simulink model "adcddcxaui_100"  (Simulink 6.2)
settings: Solver=ode45  StartTime=0.0  StopTime=1000  RelTol=1e-3
undefined symbols (not defined in the file): BitWidth
libraries: xbsIndex_r3 x358, casper_library x26, xps_library x12
(part 2 of 4)

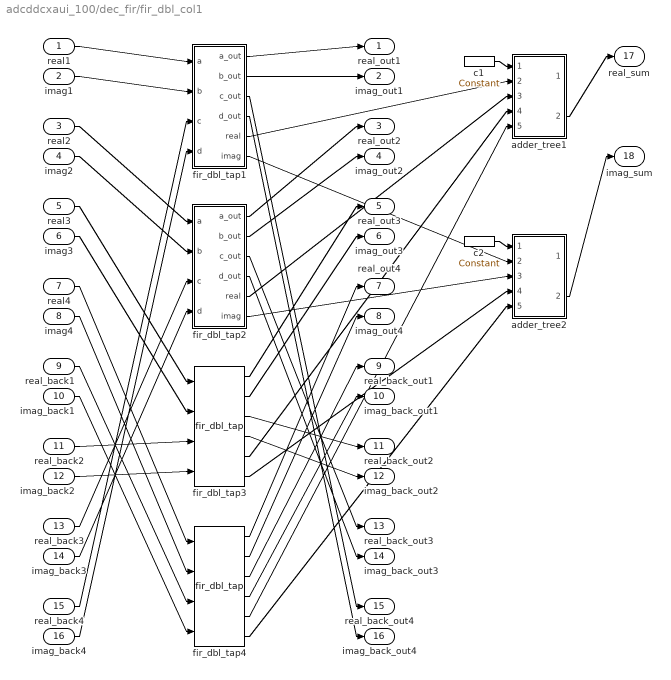
== system adcddcxaui_100/dec_fir/fir_dbl_col1 ==
  real1 : Inport  Port=1  LatchInput=off
  imag1 : Inport  Port=2  LatchInput=off
  real2 : Inport  Port=3  LatchInput=off
  imag2 : Inport  Port=4  LatchInput=off
  real3 : Inport  Port=5  LatchInput=off
  imag3 : Inport  Port=6  LatchInput=off
  real4 : Inport  Port=7  LatchInput=off
  imag4 : Inport  Port=8  LatchInput=off
  real_back1 : Inport  Port=9  LatchInput=off
  imag_back1 : Inport  Port=10  LatchInput=off
  real_back2 : Inport  Port=11  LatchInput=off
  imag_back2 : Inport  Port=12  LatchInput=off
  real_back3 : Inport  Port=13  LatchInput=off
  imag_back3 : Inport  Port=14  LatchInput=off
  real_back4 : Inport  Port=15  LatchInput=off
  imag_back4 : Inport  Port=16  LatchInput=off
  adder_tree1 : Subsystem  AncestorBlock=casper_library/Misc/adder_tree  mask(adder_tree){n_inputs=4, latency=2}
      mask prompts: n_inputs "Number of Inputs"; latency "Add Latency"
      mask help: Sums all inputs using a tree of adds and delays.
      mask init:
      | adder_tree_init(gcb, ...
      |     'n_inputs', n_inputs, ...
      |     'latency', latency);
      settings: AttributesFormatString=latency 4
      mask Help: eval('xlWeb([getenv(''MLIB_ROOT''), ''\doc\html\sp_adder_tree\sp_adder_tree.html''])')
  adder_tree2 : Subsystem  AncestorBlock=casper_library/Misc/adder_tree  mask(adder_tree){n_inputs=4, latency=2}
      mask prompts: n_inputs "Number of Inputs"; latency "Add Latency"
      mask help: Sums all inputs using a tree of adds and delays.
      mask init:
      | adder_tree_init(gcb, ...
      |     'n_inputs', n_inputs, ...
      |     'latency', latency);
      settings: AttributesFormatString=latency 4
      mask Help: eval('xlWeb([getenv(''MLIB_ROOT''), ''\doc\html\sp_adder_tree\sp_adder_tree.html''])')
  c1 : xbsIndex_r3/Constant  const=1  equ=P=C  arith_type=Unsigned  n_bits=1  bin_pt=0  opselect=C  inp2=PCIN>>17  opr=+  inp1=P  carry=CIN  iostate=0  explicit_period=on  period=1  dbl_ovrd=off
  c2 : xbsIndex_r3/Constant  const=1  equ=P=C  arith_type=Unsigned  n_bits=1  bin_pt=0  opselect=C  inp2=PCIN>>17  opr=+  inp1=P  carry=CIN  iostate=0  explicit_period=on  period=1  dbl_ovrd=off
  fir_dbl_tap1 : Subsystem  AncestorBlock=casper_library/Downconverter/fir_dbl_tap  mask(fir_dbl_tap){factor=-6.8471e-006, add_latency=2, mult_latency=2}
      mask prompts: add_latency "Add latency"; mult_latency "Mult latency"
  fir_dbl_tap2 : Subsystem  AncestorBlock=casper_library/Downconverter/fir_dbl_tap  mask(fir_dbl_tap){factor=-6.7515e-006, add_latency=2, mult_latency=2}
      mask prompts: add_latency "Add latency"; mult_latency "Mult latency"
  fir_dbl_tap3 : casper_library/Downconverter/fir_dbl_tap  factor=-1.9679e-006  add_latency=2  mult_latency=2
      link override Constant: equ=P=C
  fir_dbl_tap4 : casper_library/Downconverter/fir_dbl_tap  factor=-2.3202e-007  add_latency=2  mult_latency=2
      link override Constant: equ=P=C
  real_out1 : Outport
  imag_out1 : Outport  Port=2
  real_out2 : Outport  Port=3
  imag_out2 : Outport  Port=4
  real_out3 : Outport  Port=5
  imag_out3 : Outport  Port=6
  real_out4 : Outport  Port=7
  imag_out4 : Outport  Port=8
  real_back_out1 : Outport  Port=9
  imag_back_out1 : Outport  Port=10
  real_back_out2 : Outport  Port=11
  imag_back_out2 : Outport  Port=12
  real_back_out3 : Outport  Port=13
  imag_back_out3 : Outport  Port=14
  real_back_out4 : Outport  Port=15
  imag_back_out4 : Outport  Port=16
  real_sum : Outport  Port=17
  imag_sum : Outport  Port=18
  wires:
  c1/1 -> adder_tree1/1(sync)
  c2/1 -> adder_tree2/1(sync)
  adder_tree1/2(dout) -> real_sum/1
  adder_tree2/2(dout) -> imag_sum/1
  real1/1 -> fir_dbl_tap1/1(a)
  imag1/1 -> fir_dbl_tap1/2(b)
  real_back4/1 -> fir_dbl_tap1/3(c)
  imag_back4/1 -> fir_dbl_tap1/4(d)
  fir_dbl_tap1/1(a_out) -> real_out1/1
  fir_dbl_tap1/2(b_out) -> imag_out1/1
  fir_dbl_tap1/3(c_out) -> real_back_out4/1
  fir_dbl_tap1/4(d_out) -> imag_back_out4/1
  fir_dbl_tap1/5(real) -> adder_tree1/2(din1)
  fir_dbl_tap1/6(imag) -> adder_tree2/2(din1)
  real2/1 -> fir_dbl_tap2/1(a)
  imag2/1 -> fir_dbl_tap2/2(b)
  real_back3/1 -> fir_dbl_tap2/3(c)
  imag_back3/1 -> fir_dbl_tap2/4(d)
  fir_dbl_tap2/1(a_out) -> real_out2/1
  fir_dbl_tap2/2(b_out) -> imag_out2/1
  fir_dbl_tap2/3(c_out) -> real_back_out3/1
  fir_dbl_tap2/4(d_out) -> imag_back_out3/1
  fir_dbl_tap2/5(real) -> adder_tree1/3(din2)
  fir_dbl_tap2/6(imag) -> adder_tree2/3(din2)
  real3/1 -> fir_dbl_tap3/1
  imag3/1 -> fir_dbl_tap3/2
  real_back2/1 -> fir_dbl_tap3/3
  imag_back2/1 -> fir_dbl_tap3/4
  fir_dbl_tap3/1 -> real_out3/1
  fir_dbl_tap3/2 -> imag_out3/1
  fir_dbl_tap3/3 -> real_back_out2/1
  fir_dbl_tap3/4 -> imag_back_out2/1
  fir_dbl_tap3/5 -> adder_tree1/4(din3)
  fir_dbl_tap3/6 -> adder_tree2/4(din3)
  real4/1 -> fir_dbl_tap4/1
  imag4/1 -> fir_dbl_tap4/2
  real_back1/1 -> fir_dbl_tap4/3
  imag_back1/1 -> fir_dbl_tap4/4
  fir_dbl_tap4/1 -> real_out4/1
  fir_dbl_tap4/2 -> imag_out4/1
  fir_dbl_tap4/3 -> real_back_out1/1
  fir_dbl_tap4/4 -> imag_back_out1/1
  fir_dbl_tap4/5 -> adder_tree1/5(din4)
  fir_dbl_tap4/6 -> adder_tree2/5(din4)

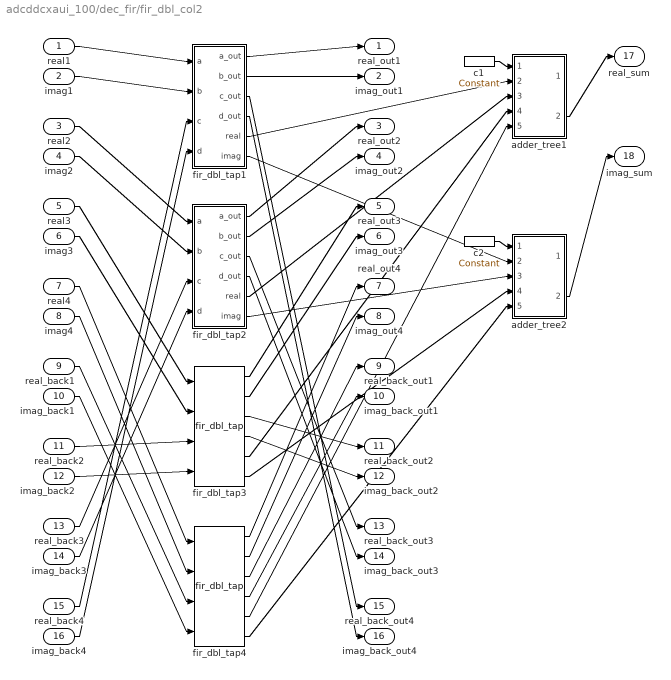
== system adcddcxaui_100/dec_fir/fir_dbl_col2 ==
  real1 : Inport  Port=1  LatchInput=off
  imag1 : Inport  Port=2  LatchInput=off
  real2 : Inport  Port=3  LatchInput=off
  imag2 : Inport  Port=4  LatchInput=off
  real3 : Inport  Port=5  LatchInput=off
  imag3 : Inport  Port=6  LatchInput=off
  real4 : Inport  Port=7  LatchInput=off
  imag4 : Inport  Port=8  LatchInput=off
  real_back1 : Inport  Port=9  LatchInput=off
  imag_back1 : Inport  Port=10  LatchInput=off
  real_back2 : Inport  Port=11  LatchInput=off
  imag_back2 : Inport  Port=12  LatchInput=off
  real_back3 : Inport  Port=13  LatchInput=off
  imag_back3 : Inport  Port=14  LatchInput=off
  real_back4 : Inport  Port=15  LatchInput=off
  imag_back4 : Inport  Port=16  LatchInput=off
  adder_tree1 : Subsystem  AncestorBlock=casper_library/Misc/adder_tree  mask(adder_tree){n_inputs=4, latency=2}
      mask prompts: n_inputs "Number of Inputs"; latency "Add Latency"
      mask help: Sums all inputs using a tree of adds and delays.
      mask init:
      | adder_tree_init(gcb, ...
      |     'n_inputs', n_inputs, ...
      |     'latency', latency);
      settings: AttributesFormatString=latency 4
      mask Help: eval('xlWeb([getenv(''MLIB_ROOT''), ''\doc\html\sp_adder_tree\sp_adder_tree.html''])')
  adder_tree2 : Subsystem  AncestorBlock=casper_library/Misc/adder_tree  mask(adder_tree){n_inputs=4, latency=2}
      mask prompts: n_inputs "Number of Inputs"; latency "Add Latency"
      mask help: Sums all inputs using a tree of adds and delays.
      mask init:
      | adder_tree_init(gcb, ...
      |     'n_inputs', n_inputs, ...
      |     'latency', latency);
      settings: AttributesFormatString=latency 4
      mask Help: eval('xlWeb([getenv(''MLIB_ROOT''), ''\doc\html\sp_adder_tree\sp_adder_tree.html''])')
  c1 : xbsIndex_r3/Constant  const=1  equ=P=C  arith_type=Unsigned  n_bits=1  bin_pt=0  opselect=C  inp2=PCIN>>17  opr=+  inp1=P  carry=CIN  iostate=0  explicit_period=on  period=1  dbl_ovrd=off
  c2 : xbsIndex_r3/Constant  const=1  equ=P=C  arith_type=Unsigned  n_bits=1  bin_pt=0  opselect=C  inp2=PCIN>>17  opr=+  inp1=P  carry=CIN  iostate=0  explicit_period=on  period=1  dbl_ovrd=off
  fir_dbl_tap1 : Subsystem  AncestorBlock=casper_library/Downconverter/fir_dbl_tap  mask(fir_dbl_tap){factor=7.4933e-005, add_latency=2, mult_latency=2}
      mask prompts: add_latency "Add latency"; mult_latency "Mult latency"
  fir_dbl_tap2 : Subsystem  AncestorBlock=casper_library/Downconverter/fir_dbl_tap  mask(fir_dbl_tap){factor=0.00010979, add_latency=2, mult_latency=2}
      mask prompts: add_latency "Add latency"; mult_latency "Mult latency"
  fir_dbl_tap3 : casper_library/Downconverter/fir_dbl_tap  factor=6.3269e-005  add_latency=2  mult_latency=2
      link override Constant: equ=P=C
  fir_dbl_tap4 : casper_library/Downconverter/fir_dbl_tap  factor=1.4095e-005  add_latency=2  mult_latency=2
      link override Constant: equ=P=C
  real_out1 : Outport
  imag_out1 : Outport  Port=2
  real_out2 : Outport  Port=3
  imag_out2 : Outport  Port=4
  real_out3 : Outport  Port=5
  imag_out3 : Outport  Port=6
  real_out4 : Outport  Port=7
  imag_out4 : Outport  Port=8
  real_back_out1 : Outport  Port=9
  imag_back_out1 : Outport  Port=10
  real_back_out2 : Outport  Port=11
  imag_back_out2 : Outport  Port=12
  real_back_out3 : Outport  Port=13
  imag_back_out3 : Outport  Port=14
  real_back_out4 : Outport  Port=15
  imag_back_out4 : Outport  Port=16
  real_sum : Outport  Port=17
  imag_sum : Outport  Port=18
  wires:
  c1/1 -> adder_tree1/1(sync)
  c2/1 -> adder_tree2/1(sync)
  adder_tree1/2(dout) -> real_sum/1
  adder_tree2/2(dout) -> imag_sum/1
  real1/1 -> fir_dbl_tap1/1(a)
  imag1/1 -> fir_dbl_tap1/2(b)
  real_back4/1 -> fir_dbl_tap1/3(c)
  imag_back4/1 -> fir_dbl_tap1/4(d)
  fir_dbl_tap1/1(a_out) -> real_out1/1
  fir_dbl_tap1/2(b_out) -> imag_out1/1
  fir_dbl_tap1/3(c_out) -> real_back_out4/1
  fir_dbl_tap1/4(d_out) -> imag_back_out4/1
  fir_dbl_tap1/5(real) -> adder_tree1/2(din1)
  fir_dbl_tap1/6(imag) -> adder_tree2/2(din1)
  real2/1 -> fir_dbl_tap2/1(a)
  imag2/1 -> fir_dbl_tap2/2(b)
  real_back3/1 -> fir_dbl_tap2/3(c)
  imag_back3/1 -> fir_dbl_tap2/4(d)
  fir_dbl_tap2/1(a_out) -> real_out2/1
  fir_dbl_tap2/2(b_out) -> imag_out2/1
  fir_dbl_tap2/3(c_out) -> real_back_out3/1
  fir_dbl_tap2/4(d_out) -> imag_back_out3/1
  fir_dbl_tap2/5(real) -> adder_tree1/3(din2)
  fir_dbl_tap2/6(imag) -> adder_tree2/3(din2)
  real3/1 -> fir_dbl_tap3/1
  imag3/1 -> fir_dbl_tap3/2
  real_back2/1 -> fir_dbl_tap3/3
  imag_back2/1 -> fir_dbl_tap3/4
  fir_dbl_tap3/1 -> real_out3/1
  fir_dbl_tap3/2 -> imag_out3/1
  fir_dbl_tap3/3 -> real_back_out2/1
  fir_dbl_tap3/4 -> imag_back_out2/1
  fir_dbl_tap3/5 -> adder_tree1/4(din3)
  fir_dbl_tap3/6 -> adder_tree2/4(din3)
  real4/1 -> fir_dbl_tap4/1
  imag4/1 -> fir_dbl_tap4/2
  real_back1/1 -> fir_dbl_tap4/3
  imag_back1/1 -> fir_dbl_tap4/4
  fir_dbl_tap4/1 -> real_out4/1
  fir_dbl_tap4/2 -> imag_out4/1
  fir_dbl_tap4/3 -> real_back_out1/1
  fir_dbl_tap4/4 -> imag_back_out1/1
  fir_dbl_tap4/5 -> adder_tree1/5(din4)
  fir_dbl_tap4/6 -> adder_tree2/5(din4)

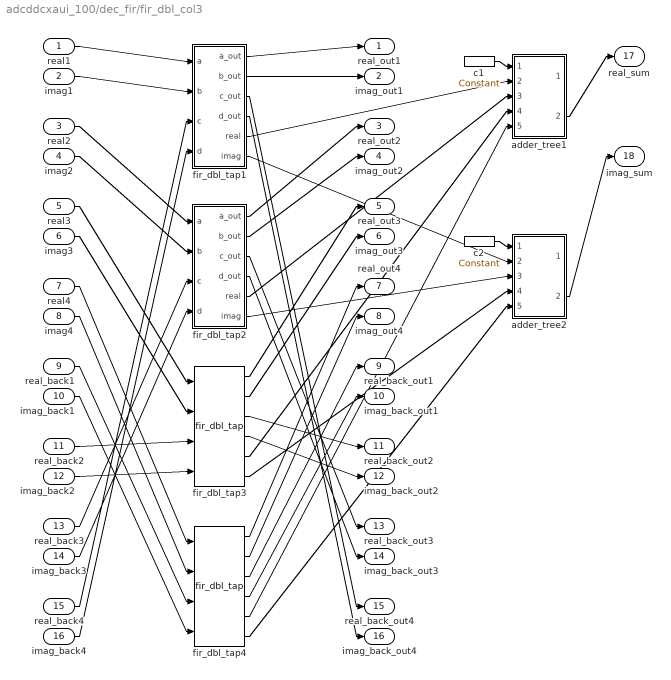
== system adcddcxaui_100/dec_fir/fir_dbl_col3 ==
  real1 : Inport  Port=1  LatchInput=off
  imag1 : Inport  Port=2  LatchInput=off
  real2 : Inport  Port=3  LatchInput=off
  imag2 : Inport  Port=4  LatchInput=off
  real3 : Inport  Port=5  LatchInput=off
  imag3 : Inport  Port=6  LatchInput=off
  real4 : Inport  Port=7  LatchInput=off
  imag4 : Inport  Port=8  LatchInput=off
  real_back1 : Inport  Port=9  LatchInput=off
  imag_back1 : Inport  Port=10  LatchInput=off
  real_back2 : Inport  Port=11  LatchInput=off
  imag_back2 : Inport  Port=12  LatchInput=off
  real_back3 : Inport  Port=13  LatchInput=off
  imag_back3 : Inport  Port=14  LatchInput=off
  real_back4 : Inport  Port=15  LatchInput=off
  imag_back4 : Inport  Port=16  LatchInput=off
  adder_tree1 : Subsystem  AncestorBlock=casper_library/Misc/adder_tree  mask(adder_tree){n_inputs=4, latency=2}
      mask prompts: n_inputs "Number of Inputs"; latency "Add Latency"
      mask help: Sums all inputs using a tree of adds and delays.
      mask init:
      | adder_tree_init(gcb, ...
      |     'n_inputs', n_inputs, ...
      |     'latency', latency);
      settings: AttributesFormatString=latency 4
      mask Help: eval('xlWeb([getenv(''MLIB_ROOT''), ''\doc\html\sp_adder_tree\sp_adder_tree.html''])')
  adder_tree2 : Subsystem  AncestorBlock=casper_library/Misc/adder_tree  mask(adder_tree){n_inputs=4, latency=2}
      mask prompts: n_inputs "Number of Inputs"; latency "Add Latency"
      mask help: Sums all inputs using a tree of adds and delays.
      mask init:
      | adder_tree_init(gcb, ...
      |     'n_inputs', n_inputs, ...
      |     'latency', latency);
      settings: AttributesFormatString=latency 4
      mask Help: eval('xlWeb([getenv(''MLIB_ROOT''), ''\doc\html\sp_adder_tree\sp_adder_tree.html''])')
  c1 : xbsIndex_r3/Constant  const=1  equ=P=C  arith_type=Unsigned  n_bits=1  bin_pt=0  opselect=C  inp2=PCIN>>17  opr=+  inp1=P  carry=CIN  iostate=0  explicit_period=on  period=1  dbl_ovrd=off
  c2 : xbsIndex_r3/Constant  const=1  equ=P=C  arith_type=Unsigned  n_bits=1  bin_pt=0  opselect=C  inp2=PCIN>>17  opr=+  inp1=P  carry=CIN  iostate=0  explicit_period=on  period=1  dbl_ovrd=off
  fir_dbl_tap1 : Subsystem  AncestorBlock=casper_library/Downconverter/fir_dbl_tap  mask(fir_dbl_tap){factor=-0.00038662, add_latency=2, mult_latency=2}
      mask prompts: add_latency "Add latency"; mult_latency "Mult latency"
  fir_dbl_tap2 : Subsystem  AncestorBlock=casper_library/Downconverter/fir_dbl_tap  mask(fir_dbl_tap){factor=-0.00064661, add_latency=2, mult_latency=2}
      mask prompts: add_latency "Add latency"; mult_latency "Mult latency"
  fir_dbl_tap3 : casper_library/Downconverter/fir_dbl_tap  factor=-0.00043644  add_latency=2  mult_latency=2
      link override Constant: equ=P=C
  fir_dbl_tap4 : casper_library/Downconverter/fir_dbl_tap  factor=-0.00011843  add_latency=2  mult_latency=2
      link override Constant: equ=P=C
  real_out1 : Outport
  imag_out1 : Outport  Port=2
  real_out2 : Outport  Port=3
  imag_out2 : Outport  Port=4
  real_out3 : Outport  Port=5
  imag_out3 : Outport  Port=6
  real_out4 : Outport  Port=7
  imag_out4 : Outport  Port=8
  real_back_out1 : Outport  Port=9
  imag_back_out1 : Outport  Port=10
  real_back_out2 : Outport  Port=11
  imag_back_out2 : Outport  Port=12
  real_back_out3 : Outport  Port=13
  imag_back_out3 : Outport  Port=14
  real_back_out4 : Outport  Port=15
  imag_back_out4 : Outport  Port=16
  real_sum : Outport  Port=17
  imag_sum : Outport  Port=18
  wires:
  c1/1 -> adder_tree1/1(sync)
  c2/1 -> adder_tree2/1(sync)
  adder_tree1/2(dout) -> real_sum/1
  adder_tree2/2(dout) -> imag_sum/1
  real1/1 -> fir_dbl_tap1/1(a)
  imag1/1 -> fir_dbl_tap1/2(b)
  real_back4/1 -> fir_dbl_tap1/3(c)
  imag_back4/1 -> fir_dbl_tap1/4(d)
  fir_dbl_tap1/1(a_out) -> real_out1/1
  fir_dbl_tap1/2(b_out) -> imag_out1/1
  fir_dbl_tap1/3(c_out) -> real_back_out4/1
  fir_dbl_tap1/4(d_out) -> imag_back_out4/1
  fir_dbl_tap1/5(real) -> adder_tree1/2(din1)
  fir_dbl_tap1/6(imag) -> adder_tree2/2(din1)
  real2/1 -> fir_dbl_tap2/1(a)
  imag2/1 -> fir_dbl_tap2/2(b)
  real_back3/1 -> fir_dbl_tap2/3(c)
  imag_back3/1 -> fir_dbl_tap2/4(d)
  fir_dbl_tap2/1(a_out) -> real_out2/1
  fir_dbl_tap2/2(b_out) -> imag_out2/1
  fir_dbl_tap2/3(c_out) -> real_back_out3/1
  fir_dbl_tap2/4(d_out) -> imag_back_out3/1
  fir_dbl_tap2/5(real) -> adder_tree1/3(din2)
  fir_dbl_tap2/6(imag) -> adder_tree2/3(din2)
  real3/1 -> fir_dbl_tap3/1
  imag3/1 -> fir_dbl_tap3/2
  real_back2/1 -> fir_dbl_tap3/3
  imag_back2/1 -> fir_dbl_tap3/4
  fir_dbl_tap3/1 -> real_out3/1
  fir_dbl_tap3/2 -> imag_out3/1
  fir_dbl_tap3/3 -> real_back_out2/1
  fir_dbl_tap3/4 -> imag_back_out2/1
  fir_dbl_tap3/5 -> adder_tree1/4(din3)
  fir_dbl_tap3/6 -> adder_tree2/4(din3)
  real4/1 -> fir_dbl_tap4/1
  imag4/1 -> fir_dbl_tap4/2
  real_back1/1 -> fir_dbl_tap4/3
  imag_back1/1 -> fir_dbl_tap4/4
  fir_dbl_tap4/1 -> real_out4/1
  fir_dbl_tap4/2 -> imag_out4/1
  fir_dbl_tap4/3 -> real_back_out1/1
  fir_dbl_tap4/4 -> imag_back_out1/1
  fir_dbl_tap4/5 -> adder_tree1/5(din4)
  fir_dbl_tap4/6 -> adder_tree2/5(din4)

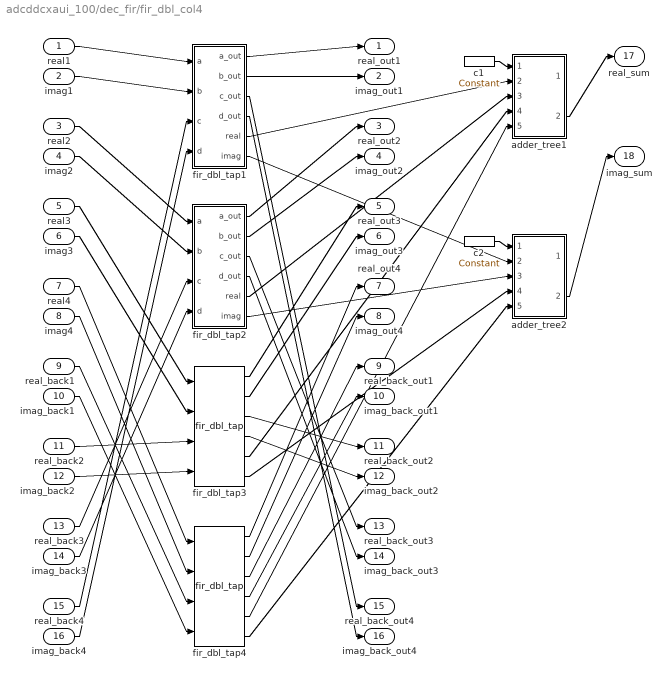
== system adcddcxaui_100/dec_fir/fir_dbl_col4 ==
  real1 : Inport  Port=1  LatchInput=off
  imag1 : Inport  Port=2  LatchInput=off
  real2 : Inport  Port=3  LatchInput=off
  imag2 : Inport  Port=4  LatchInput=off
  real3 : Inport  Port=5  LatchInput=off
  imag3 : Inport  Port=6  LatchInput=off
  real4 : Inport  Port=7  LatchInput=off
  imag4 : Inport  Port=8  LatchInput=off
  real_back1 : Inport  Port=9  LatchInput=off
  imag_back1 : Inport  Port=10  LatchInput=off
  real_back2 : Inport  Port=11  LatchInput=off
  imag_back2 : Inport  Port=12  LatchInput=off
  real_back3 : Inport  Port=13  LatchInput=off
  imag_back3 : Inport  Port=14  LatchInput=off
  real_back4 : Inport  Port=15  LatchInput=off
  imag_back4 : Inport  Port=16  LatchInput=off
  adder_tree1 : Subsystem  AncestorBlock=casper_library/Misc/adder_tree  mask(adder_tree){n_inputs=4, latency=2}
      mask prompts: n_inputs "Number of Inputs"; latency "Add Latency"
      mask help: Sums all inputs using a tree of adds and delays.
      mask init:
      | adder_tree_init(gcb, ...
      |     'n_inputs', n_inputs, ...
      |     'latency', latency);
      settings: AttributesFormatString=latency 4
      mask Help: eval('xlWeb([getenv(''MLIB_ROOT''), ''\doc\html\sp_adder_tree\sp_adder_tree.html''])')
  adder_tree2 : Subsystem  AncestorBlock=casper_library/Misc/adder_tree  mask(adder_tree){n_inputs=4, latency=2}
      mask prompts: n_inputs "Number of Inputs"; latency "Add Latency"
      mask help: Sums all inputs using a tree of adds and delays.
      mask init:
      | adder_tree_init(gcb, ...
      |     'n_inputs', n_inputs, ...
      |     'latency', latency);
      settings: AttributesFormatString=latency 4
      mask Help: eval('xlWeb([getenv(''MLIB_ROOT''), ''\doc\html\sp_adder_tree\sp_adder_tree.html''])')
  c1 : xbsIndex_r3/Constant  const=1  equ=P=C  arith_type=Unsigned  n_bits=1  bin_pt=0  opselect=C  inp2=PCIN>>17  opr=+  inp1=P  carry=CIN  iostate=0  explicit_period=on  period=1  dbl_ovrd=off
  c2 : xbsIndex_r3/Constant  const=1  equ=P=C  arith_type=Unsigned  n_bits=1  bin_pt=0  opselect=C  inp2=PCIN>>17  opr=+  inp1=P  carry=CIN  iostate=0  explicit_period=on  period=1  dbl_ovrd=off
  fir_dbl_tap1 : Subsystem  AncestorBlock=casper_library/Downconverter/fir_dbl_tap  mask(fir_dbl_tap){factor=0.0013669, add_latency=2, mult_latency=2}
      mask prompts: add_latency "Add latency"; mult_latency "Mult latency"
  fir_dbl_tap2 : Subsystem  AncestorBlock=casper_library/Downconverter/fir_dbl_tap  mask(fir_dbl_tap){factor=0.0024709, add_latency=2, mult_latency=2}
      mask prompts: add_latency "Add latency"; mult_latency "Mult latency"
  fir_dbl_tap3 : casper_library/Downconverter/fir_dbl_tap  factor=0.0018203  add_latency=2  mult_latency=2
      link override Constant: equ=P=C
  fir_dbl_tap4 : casper_library/Downconverter/fir_dbl_tap  factor=0.00054544  add_latency=2  mult_latency=2
      link override Constant: equ=P=C
  real_out1 : Outport
  imag_out1 : Outport  Port=2
  real_out2 : Outport  Port=3
  imag_out2 : Outport  Port=4
  real_out3 : Outport  Port=5
  imag_out3 : Outport  Port=6
  real_out4 : Outport  Port=7
  imag_out4 : Outport  Port=8
  real_back_out1 : Outport  Port=9
  imag_back_out1 : Outport  Port=10
  real_back_out2 : Outport  Port=11
  imag_back_out2 : Outport  Port=12
  real_back_out3 : Outport  Port=13
  imag_back_out3 : Outport  Port=14
  real_back_out4 : Outport  Port=15
  imag_back_out4 : Outport  Port=16
  real_sum : Outport  Port=17
  imag_sum : Outport  Port=18
  wires:
  c1/1 -> adder_tree1/1(sync)
  c2/1 -> adder_tree2/1(sync)
  adder_tree1/2(dout) -> real_sum/1
  adder_tree2/2(dout) -> imag_sum/1
  real1/1 -> fir_dbl_tap1/1(a)
  imag1/1 -> fir_dbl_tap1/2(b)
  real_back4/1 -> fir_dbl_tap1/3(c)
  imag_back4/1 -> fir_dbl_tap1/4(d)
  fir_dbl_tap1/1(a_out) -> real_out1/1
  fir_dbl_tap1/2(b_out) -> imag_out1/1
  fir_dbl_tap1/3(c_out) -> real_back_out4/1
  fir_dbl_tap1/4(d_out) -> imag_back_out4/1
  fir_dbl_tap1/5(real) -> adder_tree1/2(din1)
  fir_dbl_tap1/6(imag) -> adder_tree2/2(din1)
  real2/1 -> fir_dbl_tap2/1(a)
  imag2/1 -> fir_dbl_tap2/2(b)
  real_back3/1 -> fir_dbl_tap2/3(c)
  imag_back3/1 -> fir_dbl_tap2/4(d)
  fir_dbl_tap2/1(a_out) -> real_out2/1
  fir_dbl_tap2/2(b_out) -> imag_out2/1
  fir_dbl_tap2/3(c_out) -> real_back_out3/1
  fir_dbl_tap2/4(d_out) -> imag_back_out3/1
  fir_dbl_tap2/5(real) -> adder_tree1/3(din2)
  fir_dbl_tap2/6(imag) -> adder_tree2/3(din2)
  real3/1 -> fir_dbl_tap3/1
  imag3/1 -> fir_dbl_tap3/2
  real_back2/1 -> fir_dbl_tap3/3
  imag_back2/1 -> fir_dbl_tap3/4
  fir_dbl_tap3/1 -> real_out3/1
  fir_dbl_tap3/2 -> imag_out3/1
  fir_dbl_tap3/3 -> real_back_out2/1
  fir_dbl_tap3/4 -> imag_back_out2/1
  fir_dbl_tap3/5 -> adder_tree1/4(din3)
  fir_dbl_tap3/6 -> adder_tree2/4(din3)
  real4/1 -> fir_dbl_tap4/1
  imag4/1 -> fir_dbl_tap4/2
  real_back1/1 -> fir_dbl_tap4/3
  imag_back1/1 -> fir_dbl_tap4/4
  fir_dbl_tap4/1 -> real_out4/1
  fir_dbl_tap4/2 -> imag_out4/1
  fir_dbl_tap4/3 -> real_back_out1/1
  fir_dbl_tap4/4 -> imag_back_out1/1
  fir_dbl_tap4/5 -> adder_tree1/5(din4)
  fir_dbl_tap4/6 -> adder_tree2/5(din4)

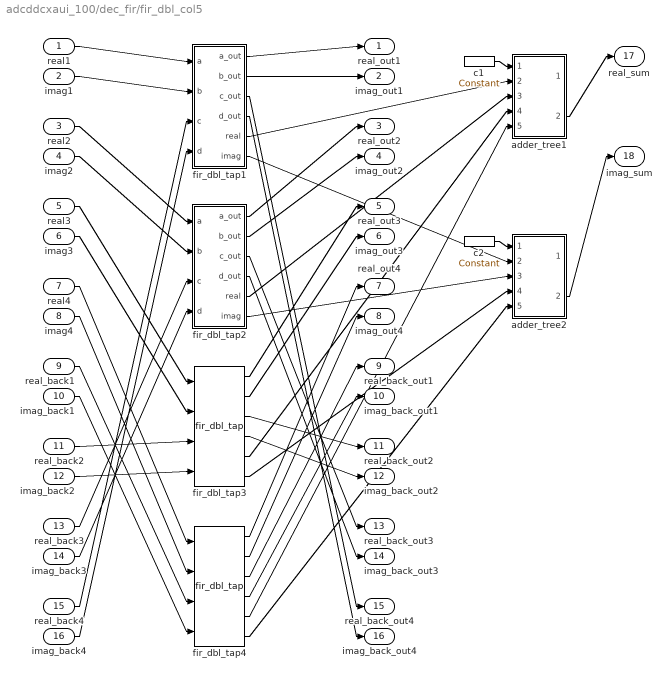
== system adcddcxaui_100/dec_fir/fir_dbl_col5 ==
  real1 : Inport  Port=1  LatchInput=off
  imag1 : Inport  Port=2  LatchInput=off
  real2 : Inport  Port=3  LatchInput=off
  imag2 : Inport  Port=4  LatchInput=off
  real3 : Inport  Port=5  LatchInput=off
  imag3 : Inport  Port=6  LatchInput=off
  real4 : Inport  Port=7  LatchInput=off
  imag4 : Inport  Port=8  LatchInput=off
  real_back1 : Inport  Port=9  LatchInput=off
  imag_back1 : Inport  Port=10  LatchInput=off
  real_back2 : Inport  Port=11  LatchInput=off
  imag_back2 : Inport  Port=12  LatchInput=off
  real_back3 : Inport  Port=13  LatchInput=off
  imag_back3 : Inport  Port=14  LatchInput=off
  real_back4 : Inport  Port=15  LatchInput=off
  imag_back4 : Inport  Port=16  LatchInput=off
  adder_tree1 : Subsystem  AncestorBlock=casper_library/Misc/adder_tree  mask(adder_tree){n_inputs=4, latency=2}
      mask prompts: n_inputs "Number of Inputs"; latency "Add Latency"
      mask help: Sums all inputs using a tree of adds and delays.
      mask init:
      | adder_tree_init(gcb, ...
      |     'n_inputs', n_inputs, ...
      |     'latency', latency);
      settings: AttributesFormatString=latency 4
      mask Help: eval('xlWeb([getenv(''MLIB_ROOT''), ''\doc\html\sp_adder_tree\sp_adder_tree.html''])')
  adder_tree2 : Subsystem  AncestorBlock=casper_library/Misc/adder_tree  mask(adder_tree){n_inputs=4, latency=2}
      mask prompts: n_inputs "Number of Inputs"; latency "Add Latency"
      mask help: Sums all inputs using a tree of adds and delays.
      mask init:
      | adder_tree_init(gcb, ...
      |     'n_inputs', n_inputs, ...
      |     'latency', latency);
      settings: AttributesFormatString=latency 4
      mask Help: eval('xlWeb([getenv(''MLIB_ROOT''), ''\doc\html\sp_adder_tree\sp_adder_tree.html''])')
  c1 : xbsIndex_r3/Constant  const=1  equ=P=C  arith_type=Unsigned  n_bits=1  bin_pt=0  opselect=C  inp2=PCIN>>17  opr=+  inp1=P  carry=CIN  iostate=0  explicit_period=on  period=1  dbl_ovrd=off
  c2 : xbsIndex_r3/Constant  const=1  equ=P=C  arith_type=Unsigned  n_bits=1  bin_pt=0  opselect=C  inp2=PCIN>>17  opr=+  inp1=P  carry=CIN  iostate=0  explicit_period=on  period=1  dbl_ovrd=off
  fir_dbl_tap1 : Subsystem  AncestorBlock=casper_library/Downconverter/fir_dbl_tap  mask(fir_dbl_tap){factor=-0.00382, add_latency=2, mult_latency=2}
      mask prompts: add_latency "Add latency"; mult_latency "Mult latency"
  fir_dbl_tap2 : Subsystem  AncestorBlock=casper_library/Downconverter/fir_dbl_tap  mask(fir_dbl_tap){factor=-0.0072503, add_latency=2, mult_latency=2}
      mask prompts: add_latency "Add latency"; mult_latency "Mult latency"
  fir_dbl_tap3 : casper_library/Downconverter/fir_dbl_tap  factor=-0.0056441  add_latency=2  mult_latency=2
      link override Constant: equ=P=C
  fir_dbl_tap4 : casper_library/Downconverter/fir_dbl_tap  factor=-0.0017992  add_latency=2  mult_latency=2
      link override Constant: equ=P=C
  real_out1 : Outport
  imag_out1 : Outport  Port=2
  real_out2 : Outport  Port=3
  imag_out2 : Outport  Port=4
  real_out3 : Outport  Port=5
  imag_out3 : Outport  Port=6
  real_out4 : Outport  Port=7
  imag_out4 : Outport  Port=8
  real_back_out1 : Outport  Port=9
  imag_back_out1 : Outport  Port=10
  real_back_out2 : Outport  Port=11
  imag_back_out2 : Outport  Port=12
  real_back_out3 : Outport  Port=13
  imag_back_out3 : Outport  Port=14
  real_back_out4 : Outport  Port=15
  imag_back_out4 : Outport  Port=16
  real_sum : Outport  Port=17
  imag_sum : Outport  Port=18
  wires:
  c1/1 -> adder_tree1/1(sync)
  c2/1 -> adder_tree2/1(sync)
  adder_tree1/2(dout) -> real_sum/1
  adder_tree2/2(dout) -> imag_sum/1
  real1/1 -> fir_dbl_tap1/1(a)
  imag1/1 -> fir_dbl_tap1/2(b)
  real_back4/1 -> fir_dbl_tap1/3(c)
  imag_back4/1 -> fir_dbl_tap1/4(d)
  fir_dbl_tap1/1(a_out) -> real_out1/1
  fir_dbl_tap1/2(b_out) -> imag_out1/1
  fir_dbl_tap1/3(c_out) -> real_back_out4/1
  fir_dbl_tap1/4(d_out) -> imag_back_out4/1
  fir_dbl_tap1/5(real) -> adder_tree1/2(din1)
  fir_dbl_tap1/6(imag) -> adder_tree2/2(din1)
  real2/1 -> fir_dbl_tap2/1(a)
  imag2/1 -> fir_dbl_tap2/2(b)
  real_back3/1 -> fir_dbl_tap2/3(c)
  imag_back3/1 -> fir_dbl_tap2/4(d)
  fir_dbl_tap2/1(a_out) -> real_out2/1
  fir_dbl_tap2/2(b_out) -> imag_out2/1
  fir_dbl_tap2/3(c_out) -> real_back_out3/1
  fir_dbl_tap2/4(d_out) -> imag_back_out3/1
  fir_dbl_tap2/5(real) -> adder_tree1/3(din2)
  fir_dbl_tap2/6(imag) -> adder_tree2/3(din2)
  real3/1 -> fir_dbl_tap3/1
  imag3/1 -> fir_dbl_tap3/2
  real_back2/1 -> fir_dbl_tap3/3
  imag_back2/1 -> fir_dbl_tap3/4
  fir_dbl_tap3/1 -> real_out3/1
  fir_dbl_tap3/2 -> imag_out3/1
  fir_dbl_tap3/3 -> real_back_out2/1
  fir_dbl_tap3/4 -> imag_back_out2/1
  fir_dbl_tap3/5 -> adder_tree1/4(din3)
  fir_dbl_tap3/6 -> adder_tree2/4(din3)
  real4/1 -> fir_dbl_tap4/1
  imag4/1 -> fir_dbl_tap4/2
  real_back1/1 -> fir_dbl_tap4/3
  imag_back1/1 -> fir_dbl_tap4/4
  fir_dbl_tap4/1 -> real_out4/1
  fir_dbl_tap4/2 -> imag_out4/1
  fir_dbl_tap4/3 -> real_back_out1/1
  fir_dbl_tap4/4 -> imag_back_out1/1
  fir_dbl_tap4/5 -> adder_tree1/5(din4)
  fir_dbl_tap4/6 -> adder_tree2/5(din4)

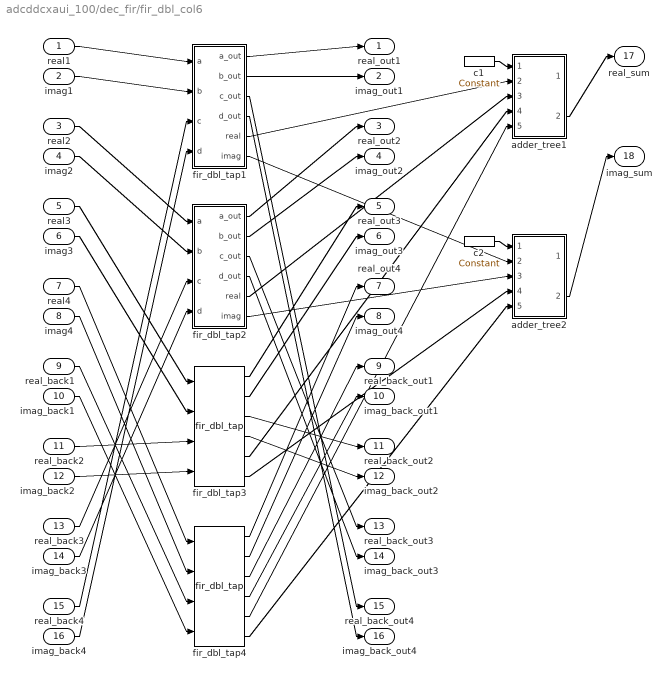
== system adcddcxaui_100/dec_fir/fir_dbl_col6 ==
  real1 : Inport  Port=1  LatchInput=off
  imag1 : Inport  Port=2  LatchInput=off
  real2 : Inport  Port=3  LatchInput=off
  imag2 : Inport  Port=4  LatchInput=off
  real3 : Inport  Port=5  LatchInput=off
  imag3 : Inport  Port=6  LatchInput=off
  real4 : Inport  Port=7  LatchInput=off
  imag4 : Inport  Port=8  LatchInput=off
  real_back1 : Inport  Port=9  LatchInput=off
  imag_back1 : Inport  Port=10  LatchInput=off
  real_back2 : Inport  Port=11  LatchInput=off
  imag_back2 : Inport  Port=12  LatchInput=off
  real_back3 : Inport  Port=13  LatchInput=off
  imag_back3 : Inport  Port=14  LatchInput=off
  real_back4 : Inport  Port=15  LatchInput=off
  imag_back4 : Inport  Port=16  LatchInput=off
  adder_tree1 : Subsystem  AncestorBlock=casper_library/Misc/adder_tree  mask(adder_tree){n_inputs=4, latency=2}
      mask prompts: n_inputs "Number of Inputs"; latency "Add Latency"
      mask help: Sums all inputs using a tree of adds and delays.
      mask init:
      | adder_tree_init(gcb, ...
      |     'n_inputs', n_inputs, ...
      |     'latency', latency);
      settings: AttributesFormatString=latency 4
      mask Help: eval('xlWeb([getenv(''MLIB_ROOT''), ''\doc\html\sp_adder_tree\sp_adder_tree.html''])')
  adder_tree2 : Subsystem  AncestorBlock=casper_library/Misc/adder_tree  mask(adder_tree){n_inputs=4, latency=2}
      mask prompts: n_inputs "Number of Inputs"; latency "Add Latency"
      mask help: Sums all inputs using a tree of adds and delays.
      mask init:
      | adder_tree_init(gcb, ...
      |     'n_inputs', n_inputs, ...
      |     'latency', latency);
      settings: AttributesFormatString=latency 4
      mask Help: eval('xlWeb([getenv(''MLIB_ROOT''), ''\doc\html\sp_adder_tree\sp_adder_tree.html''])')
  c1 : xbsIndex_r3/Constant  const=1  equ=P=C  arith_type=Unsigned  n_bits=1  bin_pt=0  opselect=C  inp2=PCIN>>17  opr=+  inp1=P  carry=CIN  iostate=0  explicit_period=on  period=1  dbl_ovrd=off
  c2 : xbsIndex_r3/Constant  const=1  equ=P=C  arith_type=Unsigned  n_bits=1  bin_pt=0  opselect=C  inp2=PCIN>>17  opr=+  inp1=P  carry=CIN  iostate=0  explicit_period=on  period=1  dbl_ovrd=off
  fir_dbl_tap1 : Subsystem  AncestorBlock=casper_library/Downconverter/fir_dbl_tap  mask(fir_dbl_tap){factor=0.0093813, add_latency=2, mult_latency=2}
      mask prompts: add_latency "Add latency"; mult_latency "Mult latency"
  fir_dbl_tap2 : Subsystem  AncestorBlock=casper_library/Downconverter/fir_dbl_tap  mask(fir_dbl_tap){factor=0.018191, add_latency=2, mult_latency=2}
      mask prompts: add_latency "Add latency"; mult_latency "Mult latency"
  fir_dbl_tap3 : casper_library/Downconverter/fir_dbl_tap  factor=0.01458  add_latency=2  mult_latency=2
      link override Constant: equ=P=C
  fir_dbl_tap4 : casper_library/Downconverter/fir_dbl_tap  factor=0.0048188  add_latency=2  mult_latency=2
      link override Constant: equ=P=C
  real_out1 : Outport
  imag_out1 : Outport  Port=2
  real_out2 : Outport  Port=3
  imag_out2 : Outport  Port=4
  real_out3 : Outport  Port=5
  imag_out3 : Outport  Port=6
  real_out4 : Outport  Port=7
  imag_out4 : Outport  Port=8
  real_back_out1 : Outport  Port=9
  imag_back_out1 : Outport  Port=10
  real_back_out2 : Outport  Port=11
  imag_back_out2 : Outport  Port=12
  real_back_out3 : Outport  Port=13
  imag_back_out3 : Outport  Port=14
  real_back_out4 : Outport  Port=15
  imag_back_out4 : Outport  Port=16
  real_sum : Outport  Port=17
  imag_sum : Outport  Port=18
  wires:
  c1/1 -> adder_tree1/1(sync)
  c2/1 -> adder_tree2/1(sync)
  adder_tree1/2(dout) -> real_sum/1
  adder_tree2/2(dout) -> imag_sum/1
  real1/1 -> fir_dbl_tap1/1(a)
  imag1/1 -> fir_dbl_tap1/2(b)
  real_back4/1 -> fir_dbl_tap1/3(c)
  imag_back4/1 -> fir_dbl_tap1/4(d)
  fir_dbl_tap1/1(a_out) -> real_out1/1
  fir_dbl_tap1/2(b_out) -> imag_out1/1
  fir_dbl_tap1/3(c_out) -> real_back_out4/1
  fir_dbl_tap1/4(d_out) -> imag_back_out4/1
  fir_dbl_tap1/5(real) -> adder_tree1/2(din1)
  fir_dbl_tap1/6(imag) -> adder_tree2/2(din1)
  real2/1 -> fir_dbl_tap2/1(a)
  imag2/1 -> fir_dbl_tap2/2(b)
  real_back3/1 -> fir_dbl_tap2/3(c)
  imag_back3/1 -> fir_dbl_tap2/4(d)
  fir_dbl_tap2/1(a_out) -> real_out2/1
  fir_dbl_tap2/2(b_out) -> imag_out2/1
  fir_dbl_tap2/3(c_out) -> real_back_out3/1
  fir_dbl_tap2/4(d_out) -> imag_back_out3/1
  fir_dbl_tap2/5(real) -> adder_tree1/3(din2)
  fir_dbl_tap2/6(imag) -> adder_tree2/3(din2)
  real3/1 -> fir_dbl_tap3/1
  imag3/1 -> fir_dbl_tap3/2
  real_back2/1 -> fir_dbl_tap3/3
  imag_back2/1 -> fir_dbl_tap3/4
  fir_dbl_tap3/1 -> real_out3/1
  fir_dbl_tap3/2 -> imag_out3/1
  fir_dbl_tap3/3 -> real_back_out2/1
  fir_dbl_tap3/4 -> imag_back_out2/1
  fir_dbl_tap3/5 -> adder_tree1/4(din3)
  fir_dbl_tap3/6 -> adder_tree2/4(din3)
  real4/1 -> fir_dbl_tap4/1
  imag4/1 -> fir_dbl_tap4/2
  real_back1/1 -> fir_dbl_tap4/3
  imag_back1/1 -> fir_dbl_tap4/4
  fir_dbl_tap4/1 -> real_out4/1
  fir_dbl_tap4/2 -> imag_out4/1
  fir_dbl_tap4/3 -> real_back_out1/1
  fir_dbl_tap4/4 -> imag_back_out1/1
  fir_dbl_tap4/5 -> adder_tree1/5(din4)
  fir_dbl_tap4/6 -> adder_tree2/5(din4)

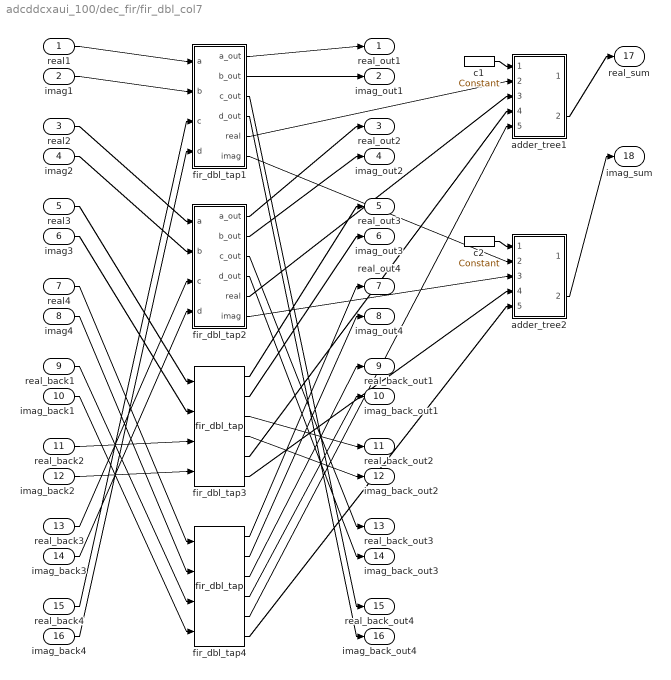
== system adcddcxaui_100/dec_fir/fir_dbl_col7 ==
  real1 : Inport  Port=1  LatchInput=off
  imag1 : Inport  Port=2  LatchInput=off
  real2 : Inport  Port=3  LatchInput=off
  imag2 : Inport  Port=4  LatchInput=off
  real3 : Inport  Port=5  LatchInput=off
  imag3 : Inport  Port=6  LatchInput=off
  real4 : Inport  Port=7  LatchInput=off
  imag4 : Inport  Port=8  LatchInput=off
  real_back1 : Inport  Port=9  LatchInput=off
  imag_back1 : Inport  Port=10  LatchInput=off
  real_back2 : Inport  Port=11  LatchInput=off
  imag_back2 : Inport  Port=12  LatchInput=off
  real_back3 : Inport  Port=13  LatchInput=off
  imag_back3 : Inport  Port=14  LatchInput=off
  real_back4 : Inport  Port=15  LatchInput=off
  imag_back4 : Inport  Port=16  LatchInput=off
  adder_tree1 : Subsystem  AncestorBlock=casper_library/Misc/adder_tree  mask(adder_tree){n_inputs=4, latency=2}
      mask prompts: n_inputs "Number of Inputs"; latency "Add Latency"
      mask help: Sums all inputs using a tree of adds and delays.
      mask init:
      | adder_tree_init(gcb, ...
      |     'n_inputs', n_inputs, ...
      |     'latency', latency);
      settings: AttributesFormatString=latency 4
      mask Help: eval('xlWeb([getenv(''MLIB_ROOT''), ''\doc\html\sp_adder_tree\sp_adder_tree.html''])')
  adder_tree2 : Subsystem  AncestorBlock=casper_library/Misc/adder_tree  mask(adder_tree){n_inputs=4, latency=2}
      mask prompts: n_inputs "Number of Inputs"; latency "Add Latency"
      mask help: Sums all inputs using a tree of adds and delays.
      mask init:
      | adder_tree_init(gcb, ...
      |     'n_inputs', n_inputs, ...
      |     'latency', latency);
      settings: AttributesFormatString=latency 4
      mask Help: eval('xlWeb([getenv(''MLIB_ROOT''), ''\doc\html\sp_adder_tree\sp_adder_tree.html''])')
  c1 : xbsIndex_r3/Constant  const=1  equ=P=C  arith_type=Unsigned  n_bits=1  bin_pt=0  opselect=C  inp2=PCIN>>17  opr=+  inp1=P  carry=CIN  iostate=0  explicit_period=on  period=1  dbl_ovrd=off
  c2 : xbsIndex_r3/Constant  const=1  equ=P=C  arith_type=Unsigned  n_bits=1  bin_pt=0  opselect=C  inp2=PCIN>>17  opr=+  inp1=P  carry=CIN  iostate=0  explicit_period=on  period=1  dbl_ovrd=off
  fir_dbl_tap1 : Subsystem  AncestorBlock=casper_library/Downconverter/fir_dbl_tap  mask(fir_dbl_tap){factor=-0.024075, add_latency=2, mult_latency=2}
      mask prompts: add_latency "Add latency"; mult_latency "Mult latency"
  fir_dbl_tap2 : Subsystem  AncestorBlock=casper_library/Downconverter/fir_dbl_tap  mask(fir_dbl_tap){factor=-0.04486, add_latency=2, mult_latency=2}
      mask prompts: add_latency "Add latency"; mult_latency "Mult latency"
  fir_dbl_tap3 : casper_library/Downconverter/fir_dbl_tap  factor=-0.035379  add_latency=2  mult_latency=2
      link override Constant: equ=P=C
  fir_dbl_tap4 : casper_library/Downconverter/fir_dbl_tap  factor=-0.011693  add_latency=2  mult_latency=2
      link override Constant: equ=P=C
  real_out1 : Outport
  imag_out1 : Outport  Port=2
  real_out2 : Outport  Port=3
  imag_out2 : Outport  Port=4
  real_out3 : Outport  Port=5
  imag_out3 : Outport  Port=6
  real_out4 : Outport  Port=7
  imag_out4 : Outport  Port=8
  real_back_out1 : Outport  Port=9
  imag_back_out1 : Outport  Port=10
  real_back_out2 : Outport  Port=11
  imag_back_out2 : Outport  Port=12
  real_back_out3 : Outport  Port=13
  imag_back_out3 : Outport  Port=14
  real_back_out4 : Outport  Port=15
  imag_back_out4 : Outport  Port=16
  real_sum : Outport  Port=17
  imag_sum : Outport  Port=18
  wires:
  c1/1 -> adder_tree1/1(sync)
  c2/1 -> adder_tree2/1(sync)
  adder_tree1/2(dout) -> real_sum/1
  adder_tree2/2(dout) -> imag_sum/1
  real1/1 -> fir_dbl_tap1/1(a)
  imag1/1 -> fir_dbl_tap1/2(b)
  real_back4/1 -> fir_dbl_tap1/3(c)
  imag_back4/1 -> fir_dbl_tap1/4(d)
  fir_dbl_tap1/1(a_out) -> real_out1/1
  fir_dbl_tap1/2(b_out) -> imag_out1/1
  fir_dbl_tap1/3(c_out) -> real_back_out4/1
  fir_dbl_tap1/4(d_out) -> imag_back_out4/1
  fir_dbl_tap1/5(real) -> adder_tree1/2(din1)
  fir_dbl_tap1/6(imag) -> adder_tree2/2(din1)
  real2/1 -> fir_dbl_tap2/1(a)
  imag2/1 -> fir_dbl_tap2/2(b)
  real_back3/1 -> fir_dbl_tap2/3(c)
  imag_back3/1 -> fir_dbl_tap2/4(d)
  fir_dbl_tap2/1(a_out) -> real_out2/1
  fir_dbl_tap2/2(b_out) -> imag_out2/1
  fir_dbl_tap2/3(c_out) -> real_back_out3/1
  fir_dbl_tap2/4(d_out) -> imag_back_out3/1
  fir_dbl_tap2/5(real) -> adder_tree1/3(din2)
  fir_dbl_tap2/6(imag) -> adder_tree2/3(din2)
  real3/1 -> fir_dbl_tap3/1
  imag3/1 -> fir_dbl_tap3/2
  real_back2/1 -> fir_dbl_tap3/3
  imag_back2/1 -> fir_dbl_tap3/4
  fir_dbl_tap3/1 -> real_out3/1
  fir_dbl_tap3/2 -> imag_out3/1
  fir_dbl_tap3/3 -> real_back_out2/1
  fir_dbl_tap3/4 -> imag_back_out2/1
  fir_dbl_tap3/5 -> adder_tree1/4(din3)
  fir_dbl_tap3/6 -> adder_tree2/4(din3)
  real4/1 -> fir_dbl_tap4/1
  imag4/1 -> fir_dbl_tap4/2
  real_back1/1 -> fir_dbl_tap4/3
  imag_back1/1 -> fir_dbl_tap4/4
  fir_dbl_tap4/1 -> real_out4/1
  fir_dbl_tap4/2 -> imag_out4/1
  fir_dbl_tap4/3 -> real_back_out1/1
  fir_dbl_tap4/4 -> imag_back_out1/1
  fir_dbl_tap4/5 -> adder_tree1/5(din4)
  fir_dbl_tap4/6 -> adder_tree2/5(din4)

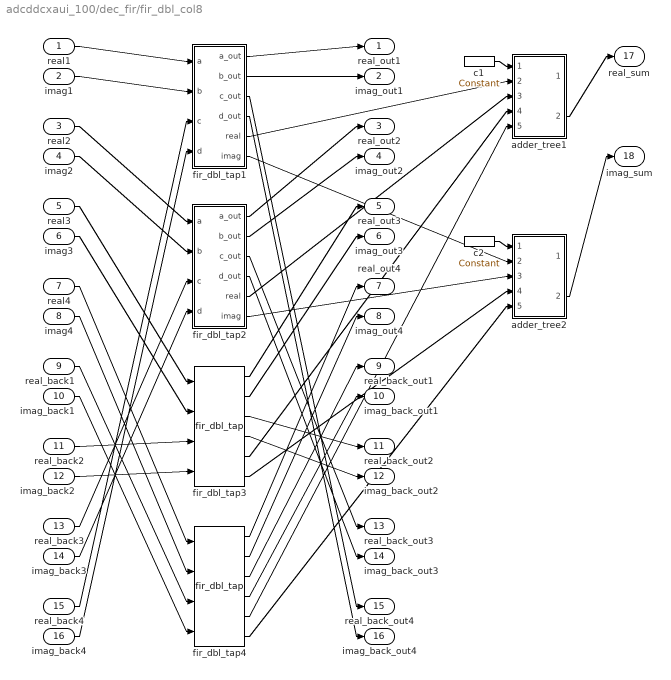
== system adcddcxaui_100/dec_fir/fir_dbl_col8 ==
  real1 : Inport  Port=1  LatchInput=off
  imag1 : Inport  Port=2  LatchInput=off
  real2 : Inport  Port=3  LatchInput=off
  imag2 : Inport  Port=4  LatchInput=off
  real3 : Inport  Port=5  LatchInput=off
  imag3 : Inport  Port=6  LatchInput=off
  real4 : Inport  Port=7  LatchInput=off
  imag4 : Inport  Port=8  LatchInput=off
  real_back1 : Inport  Port=9  LatchInput=off
  imag_back1 : Inport  Port=10  LatchInput=off
  real_back2 : Inport  Port=11  LatchInput=off
  imag_back2 : Inport  Port=12  LatchInput=off
  real_back3 : Inport  Port=13  LatchInput=off
  imag_back3 : Inport  Port=14  LatchInput=off
  real_back4 : Inport  Port=15  LatchInput=off
  imag_back4 : Inport  Port=16  LatchInput=off
  adder_tree1 : Subsystem  AncestorBlock=casper_library/Misc/adder_tree  mask(adder_tree){n_inputs=4, latency=2}
      mask prompts: n_inputs "Number of Inputs"; latency "Add Latency"
      mask help: Sums all inputs using a tree of adds and delays.
      mask init:
      | adder_tree_init(gcb, ...
      |     'n_inputs', n_inputs, ...
      |     'latency', latency);
      settings: AttributesFormatString=latency 4
      mask Help: eval('xlWeb([getenv(''MLIB_ROOT''), ''\doc\html\sp_adder_tree\sp_adder_tree.html''])')
  adder_tree2 : Subsystem  AncestorBlock=casper_library/Misc/adder_tree  mask(adder_tree){n_inputs=4, latency=2}
      mask prompts: n_inputs "Number of Inputs"; latency "Add Latency"
      mask help: Sums all inputs using a tree of adds and delays.
      mask init:
      | adder_tree_init(gcb, ...
      |     'n_inputs', n_inputs, ...
      |     'latency', latency);
      settings: AttributesFormatString=latency 4
      mask Help: eval('xlWeb([getenv(''MLIB_ROOT''), ''\doc\html\sp_adder_tree\sp_adder_tree.html''])')
  c1 : xbsIndex_r3/Constant  const=1  equ=P=C  arith_type=Unsigned  n_bits=1  bin_pt=0  opselect=C  inp2=PCIN>>17  opr=+  inp1=P  carry=CIN  iostate=0  explicit_period=on  period=1  dbl_ovrd=off
  c2 : xbsIndex_r3/Constant  const=1  equ=P=C  arith_type=Unsigned  n_bits=1  bin_pt=0  opselect=C  inp2=PCIN>>17  opr=+  inp1=P  carry=CIN  iostate=0  explicit_period=on  period=1  dbl_ovrd=off
  fir_dbl_tap1 : Subsystem  AncestorBlock=casper_library/Downconverter/fir_dbl_tap  mask(fir_dbl_tap){factor=0.24327, add_latency=2, mult_latency=2}
      mask prompts: add_latency "Add latency"; mult_latency "Mult latency"
  fir_dbl_tap2 : Subsystem  AncestorBlock=casper_library/Downconverter/fir_dbl_tap  mask(fir_dbl_tap){factor=0.19353, add_latency=2, mult_latency=2}
      mask prompts: add_latency "Add latency"; mult_latency "Mult latency"
  fir_dbl_tap3 : casper_library/Downconverter/fir_dbl_tap  factor=0.11347  add_latency=2  mult_latency=2
      link override Constant: equ=P=C
  fir_dbl_tap4 : casper_library/Downconverter/fir_dbl_tap  factor=0.032425  add_latency=2  mult_latency=2
      link override Constant: equ=P=C
  real_out1 : Outport
  imag_out1 : Outport  Port=2
  real_out2 : Outport  Port=3
  imag_out2 : Outport  Port=4
  real_out3 : Outport  Port=5
  imag_out3 : Outport  Port=6
  real_out4 : Outport  Port=7
  imag_out4 : Outport  Port=8
  real_back_out1 : Outport  Port=9
  imag_back_out1 : Outport  Port=10
  real_back_out2 : Outport  Port=11
  imag_back_out2 : Outport  Port=12
  real_back_out3 : Outport  Port=13
  imag_back_out3 : Outport  Port=14
  real_back_out4 : Outport  Port=15
  imag_back_out4 : Outport  Port=16
  real_sum : Outport  Port=17
  imag_sum : Outport  Port=18
  wires:
  c1/1 -> adder_tree1/1(sync)
  c2/1 -> adder_tree2/1(sync)
  adder_tree1/2(dout) -> real_sum/1
  adder_tree2/2(dout) -> imag_sum/1
  real1/1 -> fir_dbl_tap1/1(a)
  imag1/1 -> fir_dbl_tap1/2(b)
  real_back4/1 -> fir_dbl_tap1/3(c)
  imag_back4/1 -> fir_dbl_tap1/4(d)
  fir_dbl_tap1/1(a_out) -> real_out1/1
  fir_dbl_tap1/2(b_out) -> imag_out1/1
  fir_dbl_tap1/3(c_out) -> real_back_out4/1
  fir_dbl_tap1/4(d_out) -> imag_back_out4/1
  fir_dbl_tap1/5(real) -> adder_tree1/2(din1)
  fir_dbl_tap1/6(imag) -> adder_tree2/2(din1)
  real2/1 -> fir_dbl_tap2/1(a)
  imag2/1 -> fir_dbl_tap2/2(b)
  real_back3/1 -> fir_dbl_tap2/3(c)
  imag_back3/1 -> fir_dbl_tap2/4(d)
  fir_dbl_tap2/1(a_out) -> real_out2/1
  fir_dbl_tap2/2(b_out) -> imag_out2/1
  fir_dbl_tap2/3(c_out) -> real_back_out3/1
  fir_dbl_tap2/4(d_out) -> imag_back_out3/1
  fir_dbl_tap2/5(real) -> adder_tree1/3(din2)
  fir_dbl_tap2/6(imag) -> adder_tree2/3(din2)
  real3/1 -> fir_dbl_tap3/1
  imag3/1 -> fir_dbl_tap3/2
  real_back2/1 -> fir_dbl_tap3/3
  imag_back2/1 -> fir_dbl_tap3/4
  fir_dbl_tap3/1 -> real_out3/1
  fir_dbl_tap3/2 -> imag_out3/1
  fir_dbl_tap3/3 -> real_back_out2/1
  fir_dbl_tap3/4 -> imag_back_out2/1
  fir_dbl_tap3/5 -> adder_tree1/4(din3)
  fir_dbl_tap3/6 -> adder_tree2/4(din3)
  real4/1 -> fir_dbl_tap4/1
  imag4/1 -> fir_dbl_tap4/2
  real_back1/1 -> fir_dbl_tap4/3
  imag_back1/1 -> fir_dbl_tap4/4
  fir_dbl_tap4/1 -> real_out4/1
  fir_dbl_tap4/2 -> imag_out4/1
  fir_dbl_tap4/3 -> real_back_out1/1
  fir_dbl_tap4/4 -> imag_back_out1/1
  fir_dbl_tap4/5 -> adder_tree1/5(din4)
  fir_dbl_tap4/6 -> adder_tree2/5(din4)

== system adcddcxaui_100/dec_fir/imag_sum ==
  sync : Inport  Port=1  LatchInput=off
  din1 : Inport  Port=2  LatchInput=off
  din2 : Inport  Port=3  LatchInput=off
  din3 : Inport  Port=4  LatchInput=off
  din4 : Inport  Port=5  LatchInput=off
  din5 : Inport  Port=6  LatchInput=off
  din6 : Inport  Port=7  LatchInput=off
  din7 : Inport  Port=8  LatchInput=off
  din8 : Inport  Port=9  LatchInput=off
  addr{1..7} (7 alike) : xbsIndex_r3/AddSub  mode=Addition  precision=Full  arith_type=Unsigned  n_bits=8  bin_pt=2  quantization=Truncate  overflow=Wrap  latency=2  explicit_period=off  period=1  use_carryin=off  use_carryout=off  en=off  dbl_ovrd=off  show_param=off  use_core=on  pipeline=on  use_rpm=on  gen_core=off
      settings: xl_area=[0, 0, 0, 0, 0, 0, 0]
  sync_delay : xbsIndex_r3/Delay  latency=6  reg_retiming=off  explicit_period=off  period=1  en=off  accept_only_valid=off  init_zero=on  dbl_ovrd=off  show_param=off
      settings: xl_area=[0, 0, 0, 0, 0, 0, 0]
  sync_out : Outport
  dout : Outport  Port=2
  wires:
  addr7/1 -> dout/1
  addr6/1 -> addr7/2
  addr5/1 -> addr7/1
  addr4/1 -> addr6/2
  addr3/1 -> addr6/1
  addr2/1 -> addr5/2
  addr1/1 -> addr5/1
  din8/1 -> addr4/2
  din7/1 -> addr4/1
  din6/1 -> addr3/2
  din5/1 -> addr3/1
  din4/1 -> addr2/2
  din3/1 -> addr2/1
  din2/1 -> addr1/2
  din1/1 -> addr1/1
  sync_delay/1 -> sync_out/1
  sync/1 -> sync_delay/1

== system adcddcxaui_100/dec_fir/real_sum ==
  sync : Inport  Port=1  LatchInput=off
  din1 : Inport  Port=2  LatchInput=off
  din2 : Inport  Port=3  LatchInput=off
  din3 : Inport  Port=4  LatchInput=off
  din4 : Inport  Port=5  LatchInput=off
  din5 : Inport  Port=6  LatchInput=off
  din6 : Inport  Port=7  LatchInput=off
  din7 : Inport  Port=8  LatchInput=off
  din8 : Inport  Port=9  LatchInput=off
  addr{1..7} (7 alike) : xbsIndex_r3/AddSub  mode=Addition  precision=Full  arith_type=Unsigned  n_bits=8  bin_pt=2  quantization=Truncate  overflow=Wrap  latency=2  explicit_period=off  period=1  use_carryin=off  use_carryout=off  en=off  dbl_ovrd=off  show_param=off  use_core=on  pipeline=on  use_rpm=on  gen_core=off
      settings: xl_area=[0, 0, 0, 0, 0, 0, 0]
  sync_delay : xbsIndex_r3/Delay  latency=6  reg_retiming=off  explicit_period=off  period=1  en=off  accept_only_valid=off  init_zero=on  dbl_ovrd=off  show_param=off
      settings: xl_area=[0, 0, 0, 0, 0, 0, 0]
  sync_out : Outport
  dout : Outport  Port=2
  wires:
  addr7/1 -> dout/1
  addr6/1 -> addr7/2
  addr5/1 -> addr7/1
  addr4/1 -> addr6/2
  addr3/1 -> addr6/1
  addr2/1 -> addr5/2
  addr1/1 -> addr5/1
  din8/1 -> addr4/2
  din7/1 -> addr4/1
  din6/1 -> addr3/2
  din5/1 -> addr3/1
  din4/1 -> addr2/2
  din3/1 -> addr2/1
  din2/1 -> addr1/2
  din1/1 -> addr1/1
  sync_delay/1 -> sync_out/1
  sync/1 -> sync_delay/1

== system adcddcxaui_100/dec_fir/ri_to_c ==
  re : Inport  Port=1  LatchInput=off
  im : Inport  Port=2  LatchInput=off
  Concat : xbsIndex_r3/Concat  num_inputs=2  explicit_period=off  period=1  dbl_ovrd=off
  Reinterpret : xbsIndex_r3/Reinterpret  force_arith_type=on  arith_type=Unsigned  force_bin_pt=on  bin_pt=0  force_valid=on
  Reinterpret1 : xbsIndex_r3/Reinterpret  force_arith_type=on  arith_type=Unsigned  force_bin_pt=on  bin_pt=0  force_valid=on
  c : Outport
  wires:
  Reinterpret/1 -> Concat/1
  Reinterpret1/1 -> Concat/2
  re/1 -> Reinterpret/1
  Concat/1 -> c/1
  im/1 -> Reinterpret1/1

== system adcddcxaui_100/mixer/dds ==
  lo_const0 : casper_library/Downconverter/lo_const  n_bits=8  phase=0
      link override const: equ=P=C
      link override const1: equ=P=C
  lo_const1 : casper_library/Downconverter/lo_const  n_bits=8  phase=1.5708
      link override const: equ=P=C
      link override const1: equ=P=C
  lo_const2 : casper_library/Downconverter/lo_const  n_bits=8  phase=3.1416
      link override const: equ=P=C
      link override const1: equ=P=C
  lo_const3 : casper_library/Downconverter/lo_const  n_bits=8  phase=4.7124
      link override const: equ=P=C
      link override const1: equ=P=C
  sin0 : Outport
  cos0 : Outport  Port=2
  sin1 : Outport  Port=3
  cos1 : Outport  Port=4
  sin2 : Outport  Port=5
  cos2 : Outport  Port=6
  sin3 : Outport  Port=7
  cos3 : Outport  Port=8
  wires:
  lo_const3/2 -> cos3/1
  lo_const3/1 -> sin3/1
  lo_const2/2 -> cos2/1
  lo_const2/1 -> sin2/1
  lo_const1/2 -> cos1/1
  lo_const1/1 -> sin1/1
  lo_const0/2 -> cos0/1
  lo_const0/1 -> sin0/1

== system adcddcxaui_100/mixer/rcmult1 ==
  d : Inport  Port=1  LatchInput=off
  sin : Inport  Port=2  LatchInput=off
  cos : Inport  Port=3  LatchInput=off
  Mult : xbsIndex_r3/Mult  precision=Full  arith_type="Signed  (2's comp)"  n_bits=BitWidth  bin_pt=BitWidth-1  quantization=Truncate  overflow=Wrap  latency=latency  explicit_period=off  period=1  en=off  dbl_ovrd=off  show_param=on  mult_type=Parallel  oversample=2  use_embedded=on  pipeline=on  use_rpm=off  placement_style=Rectangular Shape  gen_core=off
      settings: xl_area=[0, 0, 0, 0, 0, 0, 0]
  Mult1 : xbsIndex_r3/Mult  precision=Full  arith_type="Signed  (2's comp)"  n_bits=BitWidth  bin_pt=BitWidth-1  quantization=Truncate  overflow=Wrap  latency=latency  explicit_period=off  period=1  en=off  dbl_ovrd=off  show_param=on  mult_type=Parallel  oversample=2  use_embedded=on  pipeline=on  use_rpm=off  placement_style=Rectangular Shape  gen_core=off
      settings: xl_area=[0, 0, 0, 0, 0, 0, 0]
  real : Outport
  imag : Outport  Port=2
  wires:
  cos/1 -> Mult/2
  sin/1 -> Mult1/2
  d/1 -> Mult/1, Mult1/1
  Mult/1 -> real/1
  Mult1/1 -> imag/1

== system adcddcxaui_100/mixer/rcmult2 ==
  d : Inport  Port=1  LatchInput=off
  sin : Inport  Port=2  LatchInput=off
  cos : Inport  Port=3  LatchInput=off
  Mult : xbsIndex_r3/Mult  precision=Full  arith_type="Signed  (2's comp)"  n_bits=BitWidth  bin_pt=BitWidth-1  quantization=Truncate  overflow=Wrap  latency=latency  explicit_period=off  period=1  en=off  dbl_ovrd=off  show_param=on  mult_type=Parallel  oversample=2  use_embedded=on  pipeline=on  use_rpm=off  placement_style=Rectangular Shape  gen_core=off
      settings: xl_area=[0, 0, 0, 0, 0, 0, 0]
  Mult1 : xbsIndex_r3/Mult  precision=Full  arith_type="Signed  (2's comp)"  n_bits=BitWidth  bin_pt=BitWidth-1  quantization=Truncate  overflow=Wrap  latency=latency  explicit_period=off  period=1  en=off  dbl_ovrd=off  show_param=on  mult_type=Parallel  oversample=2  use_embedded=on  pipeline=on  use_rpm=off  placement_style=Rectangular Shape  gen_core=off
      settings: xl_area=[0, 0, 0, 0, 0, 0, 0]
  real : Outport
  imag : Outport  Port=2
  wires:
  cos/1 -> Mult/2
  sin/1 -> Mult1/2
  d/1 -> Mult/1, Mult1/1
  Mult/1 -> real/1
  Mult1/1 -> imag/1

== system adcddcxaui_100/mixer/rcmult3 ==
  d : Inport  Port=1  LatchInput=off
  sin : Inport  Port=2  LatchInput=off
  cos : Inport  Port=3  LatchInput=off
  Mult : xbsIndex_r3/Mult  precision=Full  arith_type="Signed  (2's comp)"  n_bits=BitWidth  bin_pt=BitWidth-1  quantization=Truncate  overflow=Wrap  latency=latency  explicit_period=off  period=1  en=off  dbl_ovrd=off  show_param=on  mult_type=Parallel  oversample=2  use_embedded=on  pipeline=on  use_rpm=off  placement_style=Rectangular Shape  gen_core=off
      settings: xl_area=[0, 0, 0, 0, 0, 0, 0]
  Mult1 : xbsIndex_r3/Mult  precision=Full  arith_type="Signed  (2's comp)"  n_bits=BitWidth  bin_pt=BitWidth-1  quantization=Truncate  overflow=Wrap  latency=latency  explicit_period=off  period=1  en=off  dbl_ovrd=off  show_param=on  mult_type=Parallel  oversample=2  use_embedded=on  pipeline=on  use_rpm=off  placement_style=Rectangular Shape  gen_core=off
      settings: xl_area=[0, 0, 0, 0, 0, 0, 0]
  real : Outport
  imag : Outport  Port=2
  wires:
  cos/1 -> Mult/2
  sin/1 -> Mult1/2
  d/1 -> Mult/1, Mult1/1
  Mult/1 -> real/1
  Mult1/1 -> imag/1
